simulink model "NonLin_n10295399"  (R2019b)
settings: Solver=ode4  StartTime=0.0  StopTime=stoptime  FixedStep=h  RelTol=1e-3
values from neighbouring files (symbols this model uses):
  A = [0 1 0 0 ... (first row only)    [main_n10295399.m]
  B = [0 ... (first row only)    [main_n10295399.m]
  C = [1 0 0 0 ... (first row only)    [main_n10295399.m]
  controller_enabled = 1    [main_n10295399.m]
  G = [x_bar(1); x_bar(3)]    [main_n10295399.m]
  J = 0.0002175    [main_n10295399.m]
  K = place(A,B,p)    [main_n10295399.m]
  k = 186.3    [main_n10295399.m]
  L = 1    [main_n10295399.m]
  L_con = place(A', C', desiredPoles)'    [main_n10295399.m]
  M = 1.3608    [main_n10295399.m]
  m = 0.096    [main_n10295399.m]
  use_state_estimates = 1    [main_n10295399.m]
  x0 = [10*pi/180 0 0.1 0]'    [main_n10295399.m]
  x_bar = [0 0 0 0]'    [main_n10295399.m]
settings Model: Creator=n9182250  LastModifiedBy=don
settings DebuggingCC: ArithmeticOperatorsInVariantConditions=warning
settings SFSimCC: CustomCodeUndefinedFunction=UseInterfaceOnly

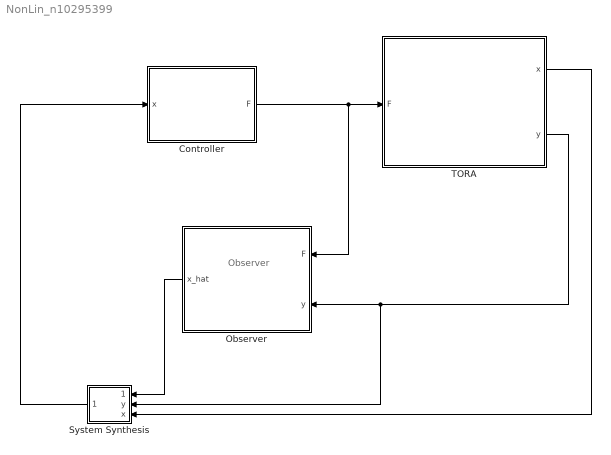
== system NonLin_n10295399 ==
  note: Observer
  Controller : Subsystem
  Observer : Subsystem
  System Synthesis : Subsystem
  TORA : Subsystem
      mask Display: image("TORA.png")
  wires:
  TORA/2(y) -> System Synthesis/2(y), Observer/2(y)
  Observer/1(x_hat) -> System Synthesis/1(x_hat)
  TORA/1(x) -> System Synthesis/3(x)
  System Synthesis/1(x_out) -> Controller/1(x)
  Controller/1(F) -> Observer/1(F), TORA/1(F)

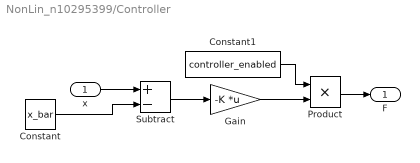
== system NonLin_n10295399/Controller ==
  x : Inport
  Constant : Constant  Value=x_bar
  Constant1 : Constant  Value=controller_enabled
  Gain : Gain  Gain=-K  Multiplication=Matrix(K*u)
  Product : Product
  Subtract : Sum  Inputs=+-
  F : Outport
  wires:
  x/1 -> Subtract/1
  Constant/1 -> Subtract/2
  Subtract/1 -> Gain/1
  Constant1/1 -> Product/1
  Gain/1 -> Product/2
  Product/1 -> F/1

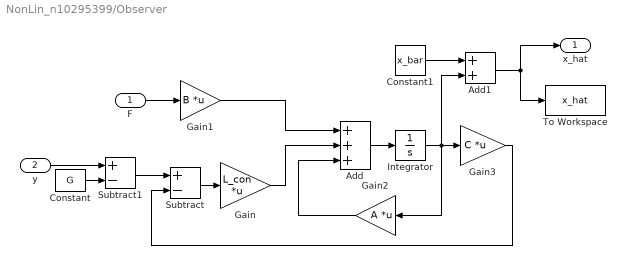
== system NonLin_n10295399/Observer ==
  F : Inport
  y : Inport  Port=2
  Add : Sum  Inputs=+++
  Add1 : Sum
  Constant : Constant  Value=G
  Constant1 : Constant  Value=x_bar
  Gain : Gain  Gain=L_con  Multiplication=Matrix(K*u)
  Gain1 : Gain  Gain=B  Multiplication=Matrix(K*u)
  Gain2 : Gain  Gain=A  Multiplication=Matrix(K*u)
  Gain3 : Gain  Gain=C  Multiplication=Matrix(K*u)
  Integrator : Integrator
  Subtract : Sum  Inputs=+-
  Subtract1 : Sum  Inputs=+-
  To Workspace : ToWorkspace  VariableName=x_hat  SampleTime=-1
  x_hat : Outport  VectorParamsAs1DForOutWhenUnconnected=off
  wires:
  Subtract/1 -> Gain/1
  F/1 -> Gain1/1
  Gain1/1 -> Add/1
  Gain/1 -> Add/2
  Add/1 -> Integrator/1
  Gain2/1 -> Add/3
  Integrator/1 -> Add1/2, Gain2/1, Gain3/1
  Gain3/1 -> Subtract/2
  y/1 -> Subtract1/1
  Subtract1/1 -> Subtract/1
  Constant/1 -> Subtract1/2
  Constant1/1 -> Add1/1
  Add1/1 -> x_hat/1, To Workspace/1

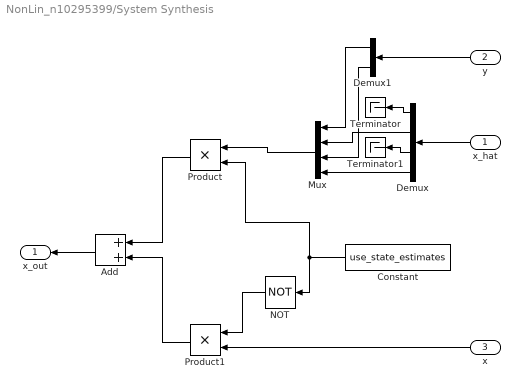
== system NonLin_n10295399/System Synthesis ==
  x_hat : Inport
  y : Inport  Port=2
  x : Inport  Port=3
  Add : Sum
  Constant : Constant  Value=use_state_estimates
  Demux : Demux
  Demux1 : Demux  Outputs=2
  Mux : Mux
  NOT : Logic  Operator=NOT  IconShape=distinctive  AllPortsSameDT=off  OutDataTypeStr=boolean
  Product : Product
  Product1 : Product
  Terminator : Terminator
  Terminator1 : Terminator
  x_out : Outport
  wires:
  x_hat/1 -> Demux/1
  Mux/1 -> Product/1
  Constant/1 -> Product/2, NOT/1
  x/1 -> Product1/2
  NOT/1 -> Product1/1
  Add/1 -> x_out/1
  Product/1 -> Add/1
  Product1/1 -> Add/2
  y/1 -> Demux1/1
  Demux/2 -> Mux/2
  Demux/4 -> Mux/4
  Demux1/1 -> Mux/1
  Demux1/2 -> Mux/3
  Demux/1 -> Terminator/1
  Demux/3 -> Terminator1/1

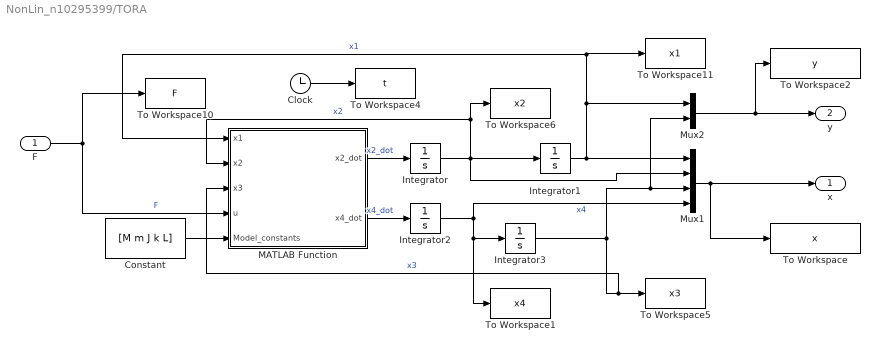
== system NonLin_n10295399/TORA ==
  F : Inport
  Clock : Clock
  Constant : Constant  Value=[M m J k L]
  Integrator : Integrator  InitialCondition=x0(2)
  Integrator1 : Integrator  InitialCondition=x0(1)
  Integrator2 : Integrator  InitialCondition=x0(4)
  Integrator3 : Integrator  InitialCondition=x0(3)
  MATLAB Function : MATLAB Function  TreatAsAtomicUnit=on
  Mux1 : Mux
  Mux2 : Mux  Inputs=2
  To Workspace : ToWorkspace  VariableName=x  SampleTime=-1
  To Workspace1 : ToWorkspace  VariableName=x4  SampleTime=-1
  To Workspace10 : ToWorkspace  VariableName=F  SampleTime=-1
  To Workspace11 : ToWorkspace  VariableName=x1  SampleTime=-1
  To Workspace2 : ToWorkspace  VariableName=y  SampleTime=-1
  To Workspace4 : ToWorkspace  VariableName=t  SampleTime=-1
  To Workspace5 : ToWorkspace  VariableName=x3  SampleTime=-1
  To Workspace6 : ToWorkspace  VariableName=x2  SampleTime=-1
  x : Outport  VectorParamsAs1DForOutWhenUnconnected=off
  y : Outport  Port=2  VectorParamsAs1DForOutWhenUnconnected=off
  wires:
  Mux1/1 -> To Workspace/1, x/1
  MATLAB Function/1(x2_dot) -> Integrator/1  "x2_dot"
  Integrator3/1 -> MATLAB Function/3(x3), To Workspace5/1, Mux2/2, Mux1/3  "x3"
  Integrator1/1 -> MATLAB Function/1(x1), To Workspace11/1, Mux2/1, Mux1/1  "x1"
  MATLAB Function/2(x4_dot) -> Integrator2/1  "x4_dot"
  Integrator/1 -> Mux1/2, To Workspace6/1, MATLAB Function/2(x2), Integrator1/1  "x2"
  F/1 -> MATLAB Function/4(u), To Workspace10/1  "F"
  Integrator2/1 -> To Workspace1/1, Integrator3/1, Mux1/4  "x4"
  Mux2/1 -> y/1, To Workspace2/1
  Constant/1 -> MATLAB Function/5(Model_constants)
  Clock/1 -> To Workspace4/1

== matlab function NonLin_n10295399/TORA/MATLAB Function ==
  data: x1 input; x2_dot output; x2 input; x3 input; u input; x4_dot output; Model_constants input
function [x2_dot,x4_dot] = NonLinearEquations(x1,x2,x3,u,Model_constants)

%Get Model Constants:
M = Model_constants(1);
m = Model_constants(2);
J = Model_constants(3);
k = Model_constants(4);
L = Model_constants(5);

%x2_dot equation
x2_dot = (((m+M)*u)-(m*L*cos(x1)*(m*L*(x2^2)*sin(x1)-(k*(x3)))))/((J+(m*(L^2))*(m+M))-((m^2)*(L^2)*cos(x1)^2));

%x4_dot equation
x4_dot = ((-m*L*u*cos(x1))+(J+(m*(L^2)))*(m*L*(x2^2)*sin(x1)-k*(x3)))/((J+(m*(L^2))*(m+M))-((m^2)*L^2*cos(x1)^2));

end
